simulink model "prima_simulazione"  (R2022b)
settings: Solver=VariableStepAuto  StartTime=0.0  StopTime=T_sim  RelTol=1e-3
values from neighbouring files (symbols this model uses):
  k = 1    [main.m]
  mu = 0.5    [main.m]
  tau = 2    [main.m]
undefined symbols (not defined in the file or in its folder): bilancia, h_max, livello_0, step_liq, step_time
settings Model: Creator=pmong  LastModifiedBy=pmong

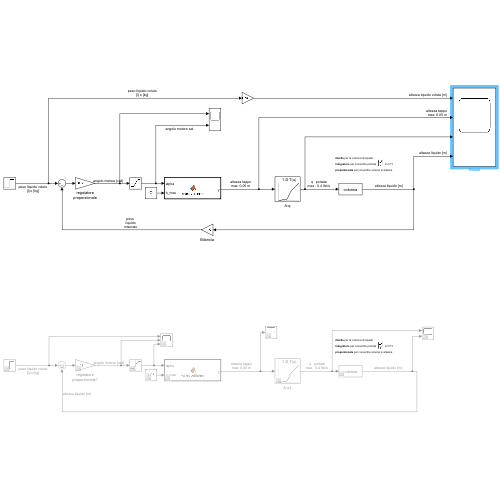
[thumbnail: Simulink's stored preview of the top-level diagram]
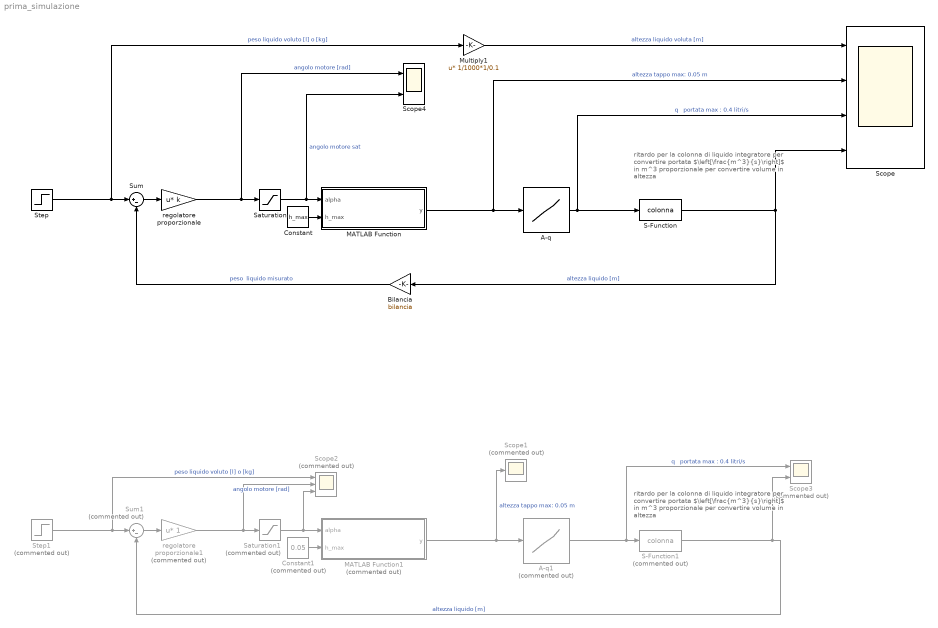
== system prima_simulazione ==
  note: ritardo per la colonna di liquido
      | integratore per convertire portata $\left[\frac{m^3}{s}\right]$ in m^3
      | proporzionale per convertire volume in altezza
  note: ritardo per la colonna di liquido
      | integratore per convertire portata $\left[\frac{m^3}{s}\right]$ in m^3
      | proporzionale per convertire volume in altezza
  A-q : Lookup_n-D  NumberOfTableDimensions=1  BreakpointsForDimension1=[0 0.005 0.01 0.015 0.02 0.025 0.03 0.035 0.04 0.045 0.05]  Table=[0 0.005 0.01 0.015 0.02 0.1 0.2 0.25 0.3 0.35 0.4]  InternalRulePriority=Speed  RndMeth=Simplest
  A-q1 : Lookup_n-D  Commented=on  NumberOfTableDimensions=1  BreakpointsForDimension1=[0 0.005 0.01 0.015 0.02 0.025 0.03 0.035 0.04 0.045 0.05]  Table=[0 0.005 0.01 0.015 0.02 0.1 0.2 0.25 0.3 0.35 0.4]  InternalRulePriority=Speed  RndMeth=Simplest
  Bilancia : Gain  Gain=bilancia
  Constant : Constant  Value=h_max
  Constant1 : Constant  Commented=on  Value=0.05
  MATLAB Function : MATLAB Function  TreatAsAtomicUnit=on
  MATLAB Function1 : MATLAB Function  Commented=on  TreatAsAtomicUnit=on
  Multiply1 : Gain  Gain=1/1000*1/0.1  Multiplication=Matrix(u*K)
  S-Function : S-Function  FunctionName=colonna  Parameters=mu,tau,livello_0  SFunctionDeploymentMode=off  EnableBusSupport=off
  S-Function1 : S-Function  Commented=on  FunctionName=colonna  Parameters=mu,tau,livello_0  SFunctionDeploymentMode=off  EnableBusSupport=off
  Saturation : Saturate  UpperLimit=pi  LowerLimit=-pi
  Saturation1 : Saturate  Commented=on  UpperLimit=pi  LowerLimit=-pi
  Scope : Scope  NumInputPorts=4
  Scope1 : Scope  Commented=on
  Scope2 : Scope  Commented=on  NumInputPorts=3
  Scope3 : Scope  Commented=on  NumInputPorts=2
  Scope4 : Scope  NumInputPorts=2
  Step : Step  Time=step_time  After=step_liq  SampleTime=0
  Step1 : Step  Commented=on  Time=5  SampleTime=0
  Sum : Sum  Inputs=|+-
  Sum1 : Sum  Commented=on  Inputs=|+-
  regolatore proporzionale : Gain  Gain=k  Multiplication=Matrix(u*K)
  regolatore proporzionale1 : Gain  Commented=on  Multiplication=Matrix(u*K)
  wires:
  Step/1 -> Sum/1, Multiply1/1  "peso liquido voluto [l] o [kg]"
  Sum/1 -> regolatore proporzionale/1
  MATLAB Function/1(y) -> Scope/2, A-q/1  "altezza tappo max: 0.05 m"
  A-q/1 -> Scope/3, S-Function/1  "q   portata max : 0.4 litri/s"
  Bilancia/1 -> Sum/2  "peso  liquido misurato"
  S-Function/1 -> Scope/4, Bilancia/1  "altezza liquido [m]"
  regolatore proporzionale/1 -> Saturation/1, Scope4/1  "angolo motore [rad]"
  Constant/1 -> MATLAB Function/2(h_max)
  Constant1/1 -> MATLAB Function1/2(h_max)
  S-Function1/1 -> Scope3/2, Sum1/2  "altezza liquido [m]"
  A-q1/1 -> Scope3/1, S-Function1/1  "q   portata max : 0.4 litri/s"
  regolatore proporzionale1/1 -> Scope2/2, Saturation1/1  "angolo motore [rad]"
  Saturation1/1 -> Scope2/3, MATLAB Function1/1(alpha)
  MATLAB Function1/1(y) -> Scope1/1, A-q1/1  "altezza tappo max: 0.05 m"
  Step1/1 -> Scope2/1, Sum1/1  "peso liquido voluto [l] o [kg]"
  Sum1/1 -> regolatore proporzionale1/1
  Saturation/1 -> Scope4/2, MATLAB Function/1(alpha)  "angolo motore sat"
  Multiply1/1 -> Scope/1  "altezza liquido voluta [m]"

== matlab function prima_simulazione/MATLAB Function ==
  data: alpha input; y output; h_max input

function y = manovellismo(alpha, h_max)
y = h_max * 0.5 *(1-cos(alpha));
end

== matlab function prima_simulazione/MATLAB Function1 ==
  data: alpha input; y output; h_max input

function y = manovellismo(alpha, h_max)
y = h_max * cos(alpha);
end
